simulink model "zad1"  (R2019b)
settings: Solver=FixedStepAuto  StartTime=0.0  StopTime=3600  FixedStep=1  RelTol=1e-3
libraries: fuzblock x3
settings Model: Creator=Avramovic  LastModifiedBy=Avramovic

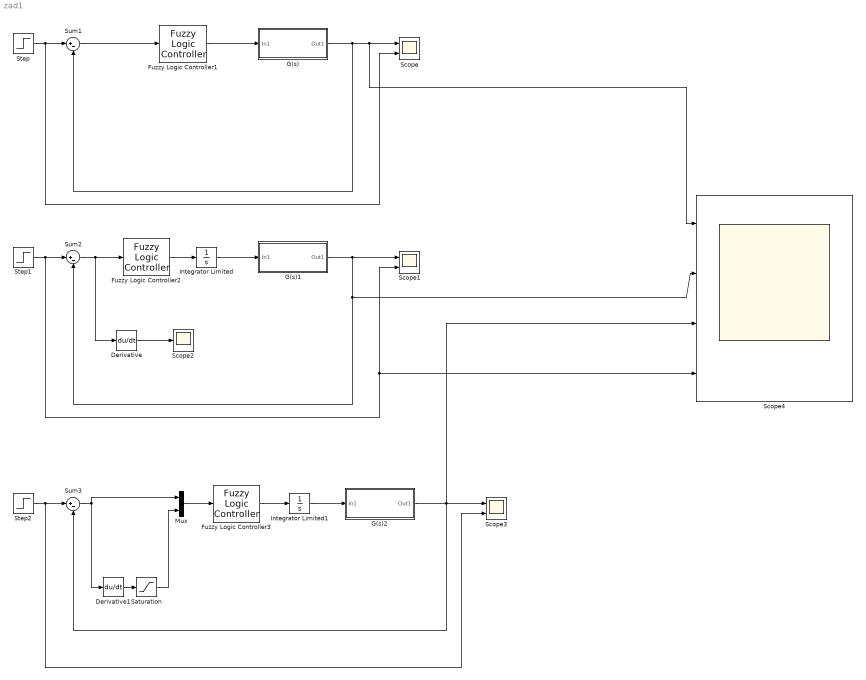
== system zad1 ==
  Derivative : Derivative
  Derivative1 : Derivative
  Fuzzy Logic Controller1 : fuzblock/Fuzzy Logic  Controller  FIS='kontr1.fis'  OutputSampleNumber=101  DataType=double  FuzzifiedInputs=off  RuleFiringStrengths=off  RuleOutputs=off  AggregatedOutputs=off  SimulateUsing=Interpreted execution  OutOfRangeInputValueMessage=warning  NoRuleFiredMessage=warning  EmptyOutputFuzzySetMessage=warning
  Fuzzy Logic Controller2 : fuzblock/Fuzzy Logic  Controller  FIS='kontr2.fis'  OutputSampleNumber=101  DataType=double  FuzzifiedInputs=off  RuleFiringStrengths=off  RuleOutputs=off  AggregatedOutputs=off  SimulateUsing=Interpreted execution  OutOfRangeInputValueMessage=warning  NoRuleFiredMessage=warning  EmptyOutputFuzzySetMessage=warning
  Fuzzy Logic Controller3 : fuzblock/Fuzzy Logic  Controller  FIS='kontr3.fis'  OutputSampleNumber=101  DataType=double  FuzzifiedInputs=off  RuleFiringStrengths=off  RuleOutputs=off  AggregatedOutputs=off  SimulateUsing=Interpreted execution  OutOfRangeInputValueMessage=warning  NoRuleFiredMessage=warning  EmptyOutputFuzzySetMessage=warning
  G(s) : Subsystem
  G(s)1 : Subsystem
  G(s)2 : Subsystem
  Integrator Limited : Integrator  LimitOutput=on  UpperSaturationLimit=1.2  LowerSaturationLimit=-1.2
  Integrator Limited1 : Integrator  LimitOutput=on  UpperSaturationLimit=1.2  LowerSaturationLimit=-1.2
  Mux : Mux  Inputs=2
  Saturation : Saturate
  Scope : Scope  NumInputPorts=2
  Scope1 : Scope  NumInputPorts=2
  Scope2 : Scope
  Scope3 : Scope  NumInputPorts=2
  Scope4 : Scope  NumInputPorts=4
  Step : Step  Time=1000  Before=-2  After=2  SampleTime=0
  Step1 : Step  Time=300  Before=-2  After=2  SampleTime=0
  Step2 : Step  Time=300  Before=-2  After=2  SampleTime=0
  Sum1 : Sum  Inputs=|+-
  Sum2 : Sum  Inputs=|+-
  Sum3 : Sum  Inputs=|+-
  wires:
  G(s)/1(Out1) -> Sum1/2, Scope4/1, Scope/1
  Step/1 -> Sum1/1, Scope/2
  Sum1/1 -> Fuzzy Logic Controller1/1
  Fuzzy Logic Controller1/1 -> G(s)/1(In1)
  G(s)1/1(Out1) -> Scope4/2, Sum2/2, Scope1/1
  Step1/1 -> Sum2/1, Scope4/4, Scope1/2
  Sum2/1 -> Derivative/1, Fuzzy Logic Controller2/1
  Fuzzy Logic Controller2/1 -> Integrator Limited/1
  Integrator Limited/1 -> G(s)1/1(In1)
  Derivative/1 -> Scope2/1
  Step2/1 -> Sum3/1, Scope3/2
  Sum3/1 -> Derivative1/1, Mux/1
  G(s)2/1(Out1) -> Scope4/3, Sum3/2, Scope3/1
  Integrator Limited1/1 -> G(s)2/1(In1)
  Fuzzy Logic Controller3/1 -> Integrator Limited1/1
  Derivative1/1 -> Saturation/1
  Mux/1 -> Fuzzy Logic Controller3/1
  Saturation/1 -> Mux/2

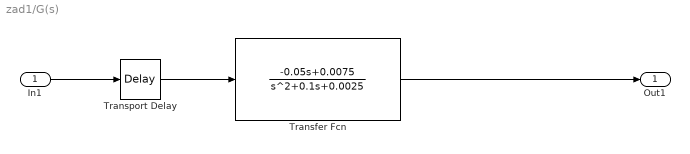
== system zad1/G(s) ==
  In1 : Inport
  Transfer Fcn : TransferFcn  Numerator=[-0.05 0.0075]  Denominator=[1 0.1 0.0025]
  Transport Delay : TransportDelay  DelayTime=3.6
  Out1 : Outport
  wires:
  In1/1 -> Transport Delay/1
  Transfer Fcn/1 -> Out1/1
  Transport Delay/1 -> Transfer Fcn/1

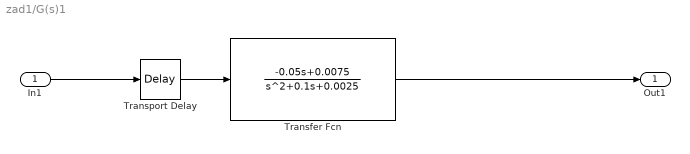
== system zad1/G(s)1 ==
  In1 : Inport
  Transfer Fcn : TransferFcn  Numerator=[-0.05 0.0075]  Denominator=[1 0.1 0.0025]
  Transport Delay : TransportDelay  DelayTime=3.6
  Out1 : Outport
  wires:
  In1/1 -> Transport Delay/1
  Transfer Fcn/1 -> Out1/1
  Transport Delay/1 -> Transfer Fcn/1

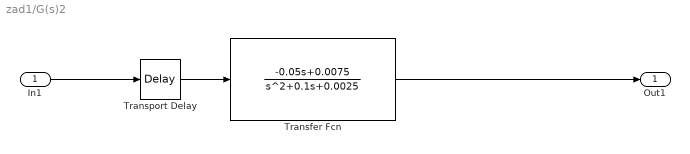
== system zad1/G(s)2 ==
  In1 : Inport
  Transfer Fcn : TransferFcn  Numerator=[-0.05 0.0075]  Denominator=[1 0.1 0.0025]
  Transport Delay : TransportDelay  DelayTime=3.6
  Out1 : Outport
  wires:
  In1/1 -> Transport Delay/1
  Transfer Fcn/1 -> Out1/1
  Transport Delay/1 -> Transfer Fcn/1
